simulink model "LUPA_Array_Eqk_circuit"  (R2024b)
settings: Solver=VariableStepAuto  StartTime=0.0  StopTime=100.0  RelTol=1e-3
undefined symbols (not defined in the file or in its folder): C_add_f1, C_add_f2, Fex_f1, Fex_f2, hydro, L_hs_f2, R_rad_f1, R_rad_f2
libraries: nesl_utility x12, fl_lib x10, ee_lib x4
settings Model: Creator=inyongkim  LastModifiedBy=inyongkim

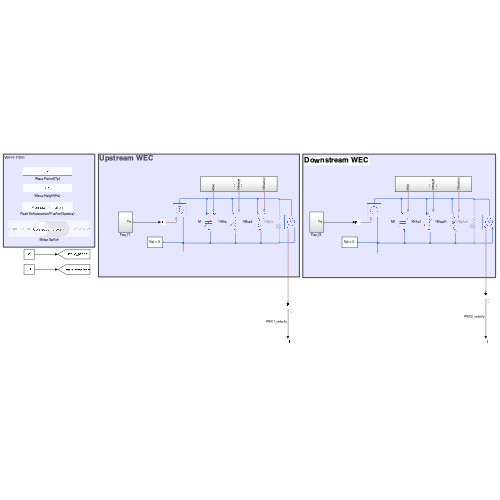
[thumbnail: Simulink's stored preview of the top-level diagram]
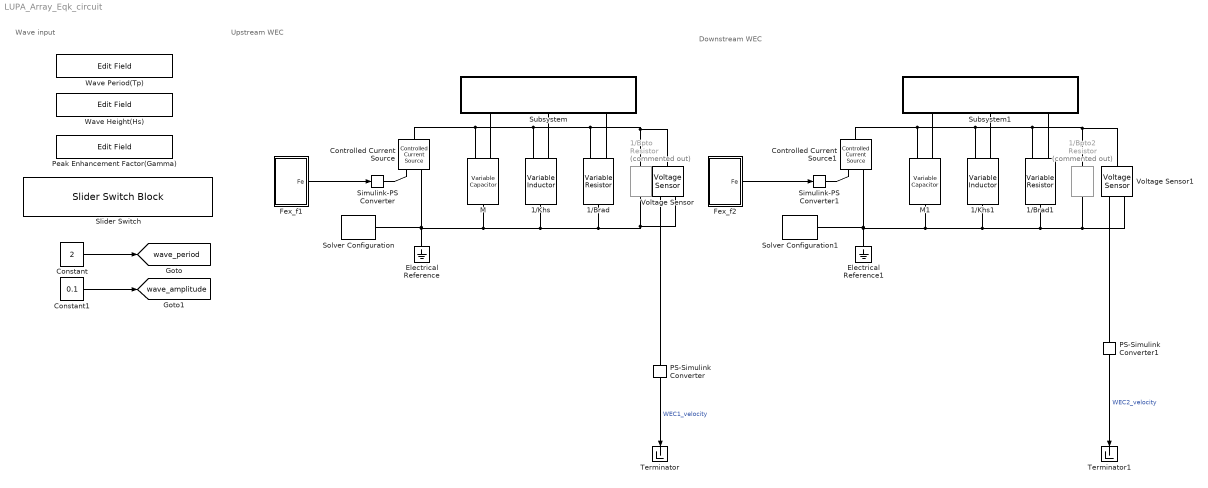
== system LUPA_Array_Eqk_circuit ==
  note: Downstream WEC
  note: Upstream WEC
  note: Wave input
  1/Bpto : fl_lib/Electrical/Electrical Elements/Resistor  Commented=on  R=1 Ohm  i_specify=off  i_priority=None  i=0 A  i_nominal_specify=off  i_nominal_value=1  i_nominal_unit=A  v_specify=off  v_priority=None  v=0 V  v_nominal_specify=off  v_nominal_value=1  v_nominal_unit=V
  1/Bpto2 : fl_lib/Electrical/Electrical Elements/Resistor  Commented=on  R=1 Ohm  i_specify=off  i_priority=None  i=0 A  i_nominal_specify=off  i_nominal_value=1  i_nominal_unit=A  v_specify=off  v_priority=None  v=0 V  v_nominal_specify=off  v_nominal_value=1  v_nominal_unit=V
  1/Brad : fl_lib/Electrical/Electrical Elements/Variable Resistor  Rmin=0 Ohm  thermalEnable=false  thermal_mass=1 J/K  i_specify=off  i_priority=None  i=0 A  i_nominal_specify=off  i_nominal_value=1  i_nominal_unit=A  v_specify=off  v_priority=None  v=0 V  v_nominal_specify=off  v_nominal_value=1  v_nominal_unit=V  T_specify=off  T_priority=None  T=300 K  T_nominal_specify=off  T_nominal_value=1  T_nominal_unit=K
  1/Brad1 : fl_lib/Electrical/Electrical Elements/Variable Resistor  Rmin=0 Ohm  thermalEnable=false  thermal_mass=1 J/K  i_specify=off  i_priority=None  i=0 A  i_nominal_specify=off  i_nominal_value=1  i_nominal_unit=A  v_specify=off  v_priority=None  v=0 V  v_nominal_specify=off  v_nominal_value=1  v_nominal_unit=V  T_specify=off  T_priority=None  T=300 K  T_nominal_specify=off  T_nominal_value=1  T_nominal_unit=K
  1/Khs : ee_lib/Passive/Variable Inductor  prm=1  Lmin=1e-6 H  g=1e-9 1/Ohm  i0=0 A  phi0=0 Wb
      settings: InternalSimscapePortConfiguration="{\"Bottom\":[],\"Left\":[{\"id\":\"L\",\"label\":\"L\",\"type\":\"input\"},{\"id\":\"p\",\"label\":\"+\",\"type\":\"foundation.electrical.electrical\"}],\"Right\":[{\"id\":\"n\",\"label\":\"-\",\"type\":\"foundation.electrical.electrical\"}],\"Top\":[]}"
  1/Khs1 : ee_lib/Passive/Variable Inductor  prm=1  Lmin=1e-6 H  g=1e-9 1/Ohm  i0=0 A  phi0=0 Wb
      settings: InternalSimscapePortConfiguration="{\"Bottom\":[],\"Left\":[{\"id\":\"L\",\"label\":\"L\",\"type\":\"input\"},{\"id\":\"p\",\"label\":\"+\",\"type\":\"foundation.electrical.electrical\"}],\"Right\":[{\"id\":\"n\",\"label\":\"-\",\"type\":\"foundation.electrical.electrical\"}],\"Top\":[]}"
  Constant : Constant  Value=2
  Constant1 : Constant  Value=0.1
  Controlled Current Source : fl_lib/Electrical/Electrical Sources/Controlled Current Source
  Controlled Current Source1 : fl_lib/Electrical/Electrical Sources/Controlled Current Source
  Electrical Reference : fl_lib/Electrical/Electrical Elements/Electrical Reference
  Electrical Reference1 : fl_lib/Electrical/Electrical Elements/Electrical Reference
  Fex_f1 : Subsystem
  Fex_f2 : Subsystem
  M : ee_lib/Passive/Variable Capacitor  prm=2  Cmin=1e-9 F  r=1e-6 Ohm  v0=0 V  q0=0 C
      settings: InternalSimscapePortConfiguration="{\"Bottom\":[],\"Left\":[{\"id\":\"C\",\"label\":\"C\",\"type\":\"input\"},{\"id\":\"p\",\"label\":\"+\",\"type\":\"foundation.electrical.electrical\"}],\"Right\":[{\"id\":\"n\",\"label\":\"-\",\"type\":\"foundation.electrical.electrical\"}],\"Top\":[]}"
  M1 : ee_lib/Passive/Variable Capacitor  prm=2  Cmin=1e-9 F  r=1e-6 Ohm  v0=0 V  q0=0 C
      settings: InternalSimscapePortConfiguration="{\"Bottom\":[],\"Left\":[{\"id\":\"C\",\"label\":\"C\",\"type\":\"input\"},{\"id\":\"p\",\"label\":\"+\",\"type\":\"foundation.electrical.electrical\"}],\"Right\":[{\"id\":\"n\",\"label\":\"-\",\"type\":\"foundation.electrical.electrical\"}],\"Top\":[]}"
  PS-Simulink Converter : nesl_utility/PS-Simulink Converter  PhysicalDomain=network_engine_domain  SubClassName=ps_output  LeftPortType=input  RightPortType=output  PseudoPeriodic=off  Frequencies=[]  VectorFormat=inherit  Unit=inherit  AffineConversion=off
  PS-Simulink Converter1 : nesl_utility/PS-Simulink Converter  PhysicalDomain=network_engine_domain  SubClassName=ps_output  LeftPortType=input  RightPortType=output  PseudoPeriodic=off  Frequencies=[]  VectorFormat=inherit  Unit=inherit  AffineConversion=off
  Peak Enhancement Factor(Gamma) : EditField  LabelPosition=Hide  ShowInitialText=on  Alignment=Center
  Simulink-PS Converter : nesl_utility/Simulink-PS Converter  PhysicalDomain=network_engine_domain  SubClassName=ps_input  LeftPortType=input  RightPortType=output  PseudoPeriodic=off  Frequencies=[]  NoiseDistribution=none  NoiseParameters=[]  Unit=A  AffineConversion=off  FilteringAndDerivatives=provide  SimscapeFilterOrder=1  InputFilterTimeConstant=0.001  UdotUserProvided=0
  Simulink-PS Converter1 : nesl_utility/Simulink-PS Converter  PhysicalDomain=network_engine_domain  SubClassName=ps_input  LeftPortType=input  RightPortType=output  PseudoPeriodic=off  Frequencies=[]  NoiseDistribution=none  NoiseParameters=[]  Unit=A  AffineConversion=off  FilteringAndDerivatives=provide  SimscapeFilterOrder=1  InputFilterTimeConstant=0.001  UdotUserProvided=0
  Slider Switch : SliderSwitchBlock  LabelPosition=Hide
      settings: Values={{'Regular Wave', 'JONSWAP'}, [0 1]}
  Solver Configuration : nesl_utility/Solver Configuration  PhysicalDomain=network_engine_domain  SubClassName=solver  LeftPortType=input  RightPortType=generic  Tones=[]  Harmonics=[]  SimulateNoise=off  Profile=off  UseLocalSampling=off  EnableSwitchedLinearOptims=on  FrequencyDomain=off  UseCCode=off  RelTol=0.001  AbsTol=0.001  MinStep=1e-09  ToWorkspace=off  RevertToSquareIcSolve=off  NumHomotopyIterations=100  PhasorMode=off  PhasorModeNumHarmonics=1  ConsistencySolver=NEWTON_XTOL_AFTER_FTOL  IndexReductionMethod=DerivativeReplacement  DoDC=off  ResidualTolerance=1e-09  ConsistencyTolSource=GLOBAL  ConsistencyAbsTol=0.001  ConsistencyRelTol=0.001  ConsistencyTolFactor=0.001  UseLocalSolver=off  LocalSolverChoice=NE_BACKWARD_EULER_ADVANCER  ResolveIndetEquations=on  FunctionEvalNumThread=1  LocalSolverSampleTime=0.001  DoFixedCost=off  MaxNonlinIter=3  MaxModeIter=2  ComputeImpulses=off  ImpulseIterations=2  LinearAlgebra=auto  LinearAlgebraNumThread=0  EquationFormulation=NE_TIME_EF  DelaysMemoryBudget=1024  AutomaticFiltering=on  FilteringTimeConstant=0.001  PartitionStorageMethod=AS_NEEDED  PartitionMemoryBudget=1024  PartitionMethod=ROBUST  MultibodyUseLocalSolver=off  MultibodyLocalSolverChoice=ODE1  MultibodyLocalSolverSampleTime=0.001
  Solver Configuration1 : nesl_utility/Solver Configuration  PhysicalDomain=network_engine_domain  SubClassName=solver  LeftPortType=input  RightPortType=generic  Tones=[]  Harmonics=[]  SimulateNoise=off  Profile=off  UseLocalSampling=off  EnableSwitchedLinearOptims=on  FrequencyDomain=off  UseCCode=off  RelTol=0.001  AbsTol=0.001  MinStep=1e-09  ToWorkspace=off  RevertToSquareIcSolve=off  NumHomotopyIterations=100  PhasorMode=off  PhasorModeNumHarmonics=1  ConsistencySolver=NEWTON_XTOL_AFTER_FTOL  IndexReductionMethod=DerivativeReplacement  DoDC=off  ResidualTolerance=1e-09  ConsistencyTolSource=GLOBAL  ConsistencyAbsTol=0.001  ConsistencyRelTol=0.001  ConsistencyTolFactor=0.001  UseLocalSolver=off  LocalSolverChoice=NE_BACKWARD_EULER_ADVANCER  ResolveIndetEquations=on  FunctionEvalNumThread=1  LocalSolverSampleTime=0.001  DoFixedCost=off  MaxNonlinIter=3  MaxModeIter=2  ComputeImpulses=off  ImpulseIterations=2  LinearAlgebra=auto  LinearAlgebraNumThread=0  EquationFormulation=NE_TIME_EF  DelaysMemoryBudget=1024  AutomaticFiltering=on  FilteringTimeConstant=0.001  PartitionStorageMethod=AS_NEEDED  PartitionMemoryBudget=1024  PartitionMethod=ROBUST  MultibodyUseLocalSolver=off  MultibodyLocalSolverChoice=ODE1  MultibodyLocalSolverSampleTime=0.001
  Subsystem : Subsystem
  Subsystem1 : Subsystem
  Terminator : Terminator
  Terminator1 : Terminator
  Voltage Sensor : fl_lib/Electrical/Electrical Sensors/Voltage Sensor
  Voltage Sensor1 : fl_lib/Electrical/Electrical Sensors/Voltage Sensor
  Wave Height(Hs) : EditField  LabelPosition=Hide  ShowInitialText=on  Alignment=Center
  Wave Period(Tp) : EditField  LabelPosition=Hide  ShowInitialText=on  Alignment=Center
  tag scope: wave_amplitude=global, wave_period=global
  wires:
  Fex_f1/1(Fe) -> Simulink-PS Converter/1
  Fex_f2/1(Fe) -> Simulink-PS Converter1/1
  PS-Simulink Converter/1 -> Terminator/1  "WEC1_velocity"
  PS-Simulink Converter1/1 -> Terminator1/1  "WEC2_velocity"
  Constant/1 -> [wave_period]
  Constant1/1 -> [wave_amplitude]
  connections:
  Controlled Current Source/LConn1 -- Voltage Sensor/LConn1 -- 1/Bpto/LConn1 -- 1/Brad/LConn2 -- 1/Khs/LConn2 -- M/LConn2
  Controlled Current Source/RConn2 -- Electrical Reference/LConn1 -- Voltage Sensor/RConn2 -- 1/Bpto/RConn1 -- 1/Brad/RConn1 -- 1/Khs/RConn1 -- M/RConn1 -- Solver Configuration/RConn1
  Simulink-PS Converter/RConn1 -- Controlled Current Source/RConn1
  Subsystem/RConn1 -- M/LConn1
  Subsystem/RConn2 -- 1/Khs/LConn1
  Subsystem/RConn3 -- 1/Brad/LConn1
  M1/RConn1 -- Voltage Sensor1/RConn2 -- 1/Bpto2/RConn1 -- 1/Brad1/RConn1 -- 1/Khs1/RConn1 -- Controlled Current Source1/RConn2 -- Solver Configuration1/RConn1 -- Electrical Reference1/LConn1
  1/Khs1/LConn2 -- Controlled Current Source1/LConn1 -- M1/LConn2 -- Voltage Sensor1/LConn1 -- 1/Bpto2/LConn1 -- 1/Brad1/LConn2
  Subsystem1/RConn3 -- 1/Brad1/LConn1
  Subsystem1/RConn1 -- M1/LConn1
  Simulink-PS Converter1/RConn1 -- Controlled Current Source1/RConn1
  Subsystem1/RConn2 -- 1/Khs1/LConn1
  Voltage Sensor/RConn1 -- PS-Simulink Converter/LConn1
  Voltage Sensor1/RConn1 -- PS-Simulink Converter1/LConn1

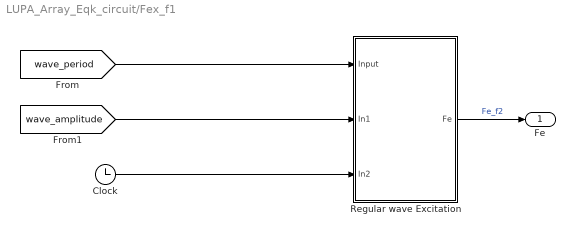
== system LUPA_Array_Eqk_circuit/Fex_f1 ==
  Clock : Clock
  Regular wave Excitation : Subsystem
  Fe : Outport
  wires:
  Regular wave Excitation/1(Fe) -> Fe/1  "Fe_f2"
  Clock/1 -> Regular wave Excitation/3(In2)
  [wave_period] -> Regular wave Excitation/1(Input)
  [wave_amplitude] -> Regular wave Excitation/2(In1)

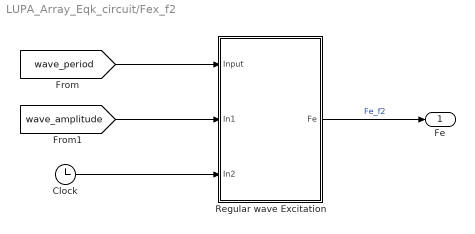
== system LUPA_Array_Eqk_circuit/Fex_f2 ==
  Clock : Clock
  Regular wave Excitation : Subsystem
  Fe : Outport
  wires:
  Regular wave Excitation/1(Fe) -> Fe/1  "Fe_f2"
  Clock/1 -> Regular wave Excitation/3(In2)
  [wave_amplitude] -> Regular wave Excitation/2(In1)
  [wave_period] -> Regular wave Excitation/1(Input)

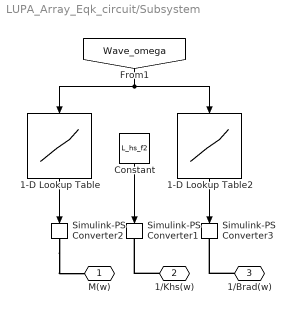
== system LUPA_Array_Eqk_circuit/Subsystem ==
  1-D Lookup Table : Lookup_n-D  NumberOfTableDimensions=1  BreakpointsForDimension1=hydro.w  Table=C_add_f1  InternalRulePriority=Speed  RndMeth=Simplest
  1-D Lookup Table2 : Lookup_n-D  NumberOfTableDimensions=1  BreakpointsForDimension1=hydro.w  Table=R_rad_f1  InternalRulePriority=Speed  RndMeth=Simplest
  Constant : Constant  Value=L_hs_f2
  Simulink-PS Converter1 : nesl_utility/Simulink-PS Converter  PhysicalDomain=network_engine_domain  SubClassName=ps_input  LeftPortType=input  RightPortType=output  PseudoPeriodic=off  Frequencies=[]  NoiseDistribution=none  NoiseParameters=[]  Unit=1  AffineConversion=off  FilteringAndDerivatives=provide  SimscapeFilterOrder=1  InputFilterTimeConstant=0.001  UdotUserProvided=0
  Simulink-PS Converter2 : nesl_utility/Simulink-PS Converter  PhysicalDomain=network_engine_domain  SubClassName=ps_input  LeftPortType=input  RightPortType=output  PseudoPeriodic=off  Frequencies=[]  NoiseDistribution=none  NoiseParameters=[]  Unit=1  AffineConversion=off  FilteringAndDerivatives=provide  SimscapeFilterOrder=1  InputFilterTimeConstant=0.001  UdotUserProvided=0
  Simulink-PS Converter3 : nesl_utility/Simulink-PS Converter  PhysicalDomain=network_engine_domain  SubClassName=ps_input  LeftPortType=input  RightPortType=output  PseudoPeriodic=off  Frequencies=[]  NoiseDistribution=none  NoiseParameters=[]  Unit=1  AffineConversion=off  FilteringAndDerivatives=provide  SimscapeFilterOrder=1  InputFilterTimeConstant=0.001  UdotUserProvided=0
  M(w) : PMIOPort  Side=Right
  1/Khs(w) : PMIOPort  Port=2  Side=Right
  1/Brad(w) : PMIOPort  Port=3  Side=Right
  wires:
  1-D Lookup Table/1 -> Simulink-PS Converter2/1
  [Wave_omega] -> 1-D Lookup Table2/1, 1-D Lookup Table/1
  1-D Lookup Table2/1 -> Simulink-PS Converter3/1
  Constant/1 -> Simulink-PS Converter1/1
  connections:
  1/Brad(w)/RConn1 -- Simulink-PS Converter3/RConn1
  1/Khs(w)/RConn1 -- Simulink-PS Converter1/RConn1
  Simulink-PS Converter2/RConn1 -- M(w)/RConn1

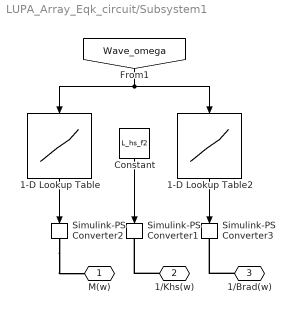
== system LUPA_Array_Eqk_circuit/Subsystem1 ==
  1-D Lookup Table : Lookup_n-D  NumberOfTableDimensions=1  BreakpointsForDimension1=hydro.w  Table=C_add_f2  InternalRulePriority=Speed  RndMeth=Simplest
  1-D Lookup Table2 : Lookup_n-D  NumberOfTableDimensions=1  BreakpointsForDimension1=hydro.w  Table=R_rad_f2  InternalRulePriority=Speed  RndMeth=Simplest
  Constant : Constant  Value=L_hs_f2
  Simulink-PS Converter1 : nesl_utility/Simulink-PS Converter  PhysicalDomain=network_engine_domain  SubClassName=ps_input  LeftPortType=input  RightPortType=output  PseudoPeriodic=off  Frequencies=[]  NoiseDistribution=none  NoiseParameters=[]  Unit=1  AffineConversion=off  FilteringAndDerivatives=provide  SimscapeFilterOrder=1  InputFilterTimeConstant=0.001  UdotUserProvided=0
  Simulink-PS Converter2 : nesl_utility/Simulink-PS Converter  PhysicalDomain=network_engine_domain  SubClassName=ps_input  LeftPortType=input  RightPortType=output  PseudoPeriodic=off  Frequencies=[]  NoiseDistribution=none  NoiseParameters=[]  Unit=1  AffineConversion=off  FilteringAndDerivatives=provide  SimscapeFilterOrder=1  InputFilterTimeConstant=0.001  UdotUserProvided=0
  Simulink-PS Converter3 : nesl_utility/Simulink-PS Converter  PhysicalDomain=network_engine_domain  SubClassName=ps_input  LeftPortType=input  RightPortType=output  PseudoPeriodic=off  Frequencies=[]  NoiseDistribution=none  NoiseParameters=[]  Unit=1  AffineConversion=off  FilteringAndDerivatives=provide  SimscapeFilterOrder=1  InputFilterTimeConstant=0.001  UdotUserProvided=0
  M(w) : PMIOPort  Side=Right
  1/Khs(w) : PMIOPort  Port=2  Side=Right
  1/Brad(w) : PMIOPort  Port=3  Side=Right
  wires:
  [Wave_omega] -> 1-D Lookup Table2/1, 1-D Lookup Table/1
  1-D Lookup Table/1 -> Simulink-PS Converter2/1
  Constant/1 -> Simulink-PS Converter1/1
  1-D Lookup Table2/1 -> Simulink-PS Converter3/1
  connections:
  1/Brad(w)/RConn1 -- Simulink-PS Converter3/RConn1
  1/Khs(w)/RConn1 -- Simulink-PS Converter1/RConn1
  Simulink-PS Converter2/RConn1 -- M(w)/RConn1

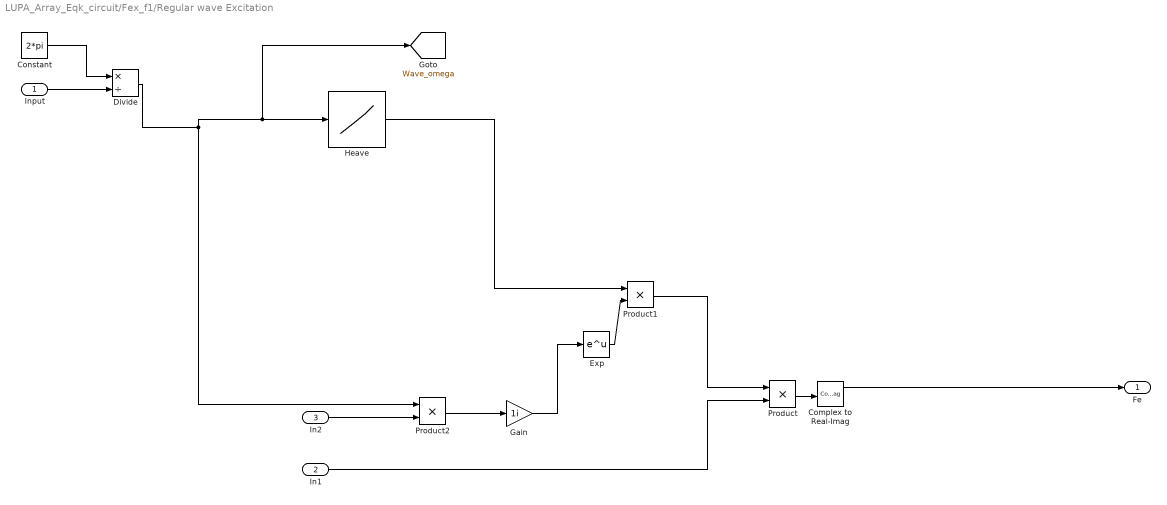
== system LUPA_Array_Eqk_circuit/Fex_f1/Regular wave Excitation ==
  Input : Inport
  In1 : Inport  Port=2
  In2 : Inport  Port=3
  Complex to Real-Imag : ComplexToRealImag
  Constant : Constant  Value=2*pi
  Divide : Product  Inputs=*/
  Exp : Math
  Gain : Gain  Gain=1i
  Heave : Lookup_n-D  NumberOfTableDimensions=1  BreakpointsForDimension1=hydro.w  Table=Fex_f1(3,:)  InternalRulePriority=Speed  RndMeth=Simplest
  Product : Product
  Product1 : Product
  Product2 : Product
  Fe : Outport
  tag scope: Wave_omega=global
  wires:
  Complex to Real-Imag/1 -> Fe/1
  Divide/1 -> [Wave_omega], Heave/1, Product2/1
  Product1/1 -> Product/1
  In1/1 -> Product/2
  In2/1 -> Product2/2
  Product2/1 -> Gain/1
  Gain/1 -> Exp/1
  Exp/1 -> Product1/2
  Product/1 -> Complex to Real-Imag/1
  Heave/1 -> Product1/1
  Input/1 -> Divide/2
  Constant/1 -> Divide/1

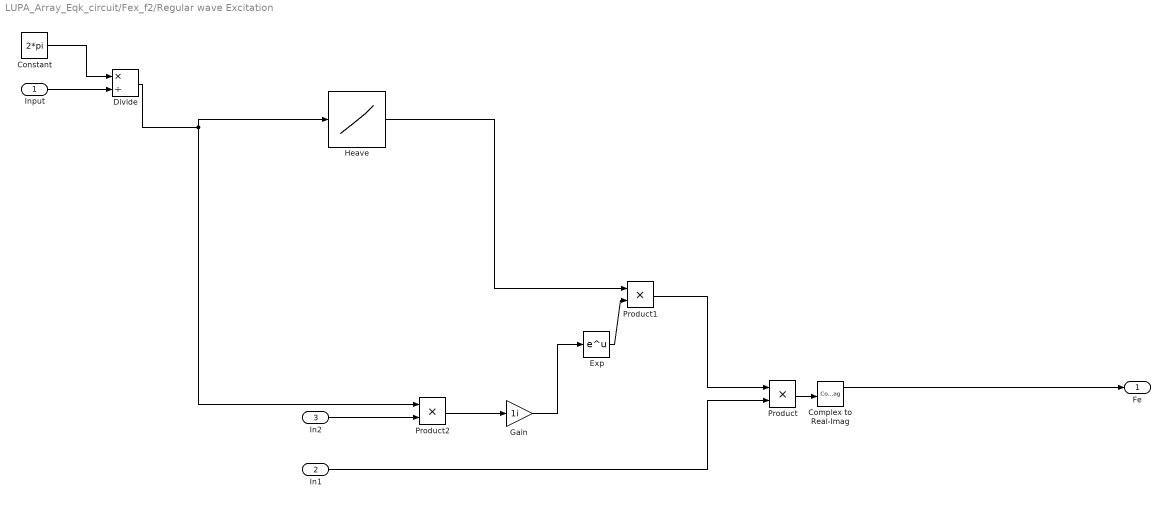
== system LUPA_Array_Eqk_circuit/Fex_f2/Regular wave Excitation ==
  Input : Inport
  In1 : Inport  Port=2
  In2 : Inport  Port=3
  Complex to Real-Imag : ComplexToRealImag
  Constant : Constant  Value=2*pi
  Divide : Product  Inputs=*/
  Exp : Math
  Gain : Gain  Gain=1i
  Heave : Lookup_n-D  NumberOfTableDimensions=1  BreakpointsForDimension1=hydro.w  Table=Fex_f2(3,:)  InternalRulePriority=Speed  RndMeth=Simplest
  Product : Product
  Product1 : Product
  Product2 : Product
  Fe : Outport
  wires:
  Complex to Real-Imag/1 -> Fe/1
  Divide/1 -> Heave/1, Product2/1
  Product1/1 -> Product/1
  In1/1 -> Product/2
  In2/1 -> Product2/2
  Product2/1 -> Gain/1
  Gain/1 -> Exp/1
  Exp/1 -> Product1/2
  Product/1 -> Complex to Real-Imag/1
  Heave/1 -> Product1/1
  Input/1 -> Divide/2
  Constant/1 -> Divide/1
